simulink model "probsix"  (Simulink 6.6)
settings: Solver=ode45  StartTime=0.0  StopTime=20.0  RelTol=1e-3
values from neighbouring files (symbols this model uses):
  Ap = r-((2*r*xe)/k)-q*upe    (= -0.1125084)    [Midterm.m]
  Bp = -q*xe    (= -11.25042)    [Midterm.m]
  g = -8    [Midterm.m]
  k = 100    [Midterm.m]
  q = 0.3    [Midterm.m]
  r = 0.3    [Midterm.m]
  upe = 0.6250    (= 0.625)    [Midterm.m]
  xe = 37.5014    [Midterm.m]
  xo = 18.75    [Midterm.m]
  z = 0.5    [Midterm.m]
settings Model: Creator=Jose  LastModifiedBy=Jose
settings DebuggingCC: SignalResolutionControl=TryResolveAllWithWarning  SolverPrmCheckMsg=none  MultiTaskDSMMsg=warning  MultiTaskCondExecSysMsg=none  StrictBusMsg=None
settings RTWCC: IncludeERTFirstTime=on

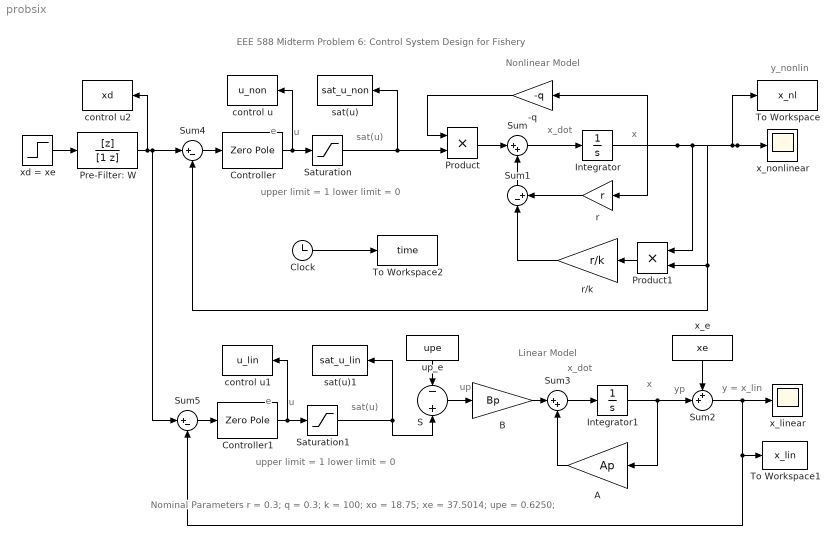
== system probsix ==
  note: Linear Model
  note: Nonlinear Model
  note: y = x_lin
  note: yp
  note: up
  note: e
  note: u
  note: upper limit = 1
      | lower limit = 0
  note: EEE 588
      | Midterm
      | Problem 6: Control System Design for Fishery
  note: x
  note: x_dot
  note: x
  note: x_dot
  note: sat(u)
  note: Nominal Parameters
      | r = 0.3; q = 0.3; k = 100; xo = 18.75; xe = 37.5014; upe = 0.6250;
  note: y_nonlin
  note: e
  note: u
  note: upper limit = 1
      | lower limit = 0
  note: sat(u)
  -q : Gain  Orientation=left  Gain=-q
  A : Gain  Orientation=left  Gain=Ap
  B : Gain  Gain=Bp
  Clock : Clock
      settings: Decimation=10
  Controller : ZeroPole  Zeros=[-z]  Poles=[0]  Gain=[g]
  Controller1 : ZeroPole  Zeros=[-z]  Poles=[0]  Gain=[g]
  Integrator : Integrator  InitialCondition=xo
  Integrator1 : Integrator  InitialCondition=xo-xe
  Pre-Filter: W : TransferFcn  Numerator=[z]  Denominator=[1 z]
  Product : Product  RndMeth=Zero
  Product1 : Product  Orientation=left  RndMeth=Zero
  S : Sum  Inputs=-+  OutScaling=2^-10
  Saturation : Saturate  UpperLimit=1  LowerLimit=0
  Saturation1 : Saturate  UpperLimit=1  LowerLimit=0
  Sum : Sum  Inputs=|++
  Sum1 : Sum  Orientation=up  Inputs=|-+
  Sum2 : Sum  Inputs=++|
  Sum3 : Sum  Inputs=|++
  Sum4 : Sum  Inputs=|+-
  Sum5 : Sum  Inputs=|+-
  To Workspace : ToWorkspace  VariableName=x_nl  SampleTime=-1  SaveFormat=Array
  To Workspace1 : ToWorkspace  VariableName=x_lin  SampleTime=-1  SaveFormat=Array
  To Workspace2 : ToWorkspace  VariableName=time  SampleTime=-1  SaveFormat=Array
  control u : ToWorkspace  VariableName=u_non  SampleTime=-1  SaveFormat=Array
  control u1 : ToWorkspace  VariableName=u_lin  SampleTime=-1  SaveFormat=Array
  control u2 : ToWorkspace  VariableName=xd  SampleTime=-1  SaveFormat=Array
  r : Gain  Orientation=left  Gain=r
  r/k : Gain  Orientation=left  Gain=r/k
  sat(u) : ToWorkspace  VariableName=sat_u_non  SampleTime=-1  SaveFormat=Array
  sat(u)1 : ToWorkspace  VariableName=sat_u_lin  SampleTime=-1  SaveFormat=Array
  up_e : Constant  Orientation=down  Value=upe
  x_e : Constant  Orientation=down  Value=xe
  x_linear : Scope
  x_nonlinear : Scope
  xd = xe : Step  Time=0  After=xe  SampleTime=0
  wires:
  Product/1 -> Sum/1
  Sum/1 -> Integrator/1
  Integrator/1 -> r/1, -q/1, Product1/1, x_nonlinear/1, Product1/2, Sum4/2, To Workspace/1
  -q/1 -> Product/1
  r/1 -> Sum1/2
  Sum1/1 -> Sum/2
  Product1/1 -> r/k/1
  r/k/1 -> Sum1/1
  Integrator1/1 -> Sum2/2, A/1
  Sum2/1 -> x_linear/1, To Workspace1/1, Sum5/2
  Sum3/1 -> Integrator1/1
  A/1 -> Sum3/2
  B/1 -> Sum3/1
  Clock/1 -> To Workspace2/1
  x_e/1 -> Sum2/1
  S/1 -> B/1
  Sum4/1 -> Controller/1
  Pre-Filter: W/1 -> Sum4/1, Sum5/1, control u2/1
  Saturation/1 -> Product/2, sat(u)/1
  Controller/1 -> Saturation/1, control u/1
  xd = xe/1 -> Pre-Filter: W/1
  up_e/1 -> S/1
  Saturation1/1 -> sat(u)1/1, S/2
  Controller1/1 -> Saturation1/1, control u1/1
  Sum5/1 -> Controller1/1
